simulink model "projeto_SOGI_PLL"  (R2018a)
settings: Solver=ode4  StartTime=0.0  StopTime=1  FixedStep=1e-4  RelTol=1e-3
undefined symbols (not defined in the file): Ibase, L, R, Vdc, Vp
libraries: powerlib_meascontrol x3, peTransforms x1
settings Model: Creator=lucas.figueiredo  LastModifiedBy=lucas.figueiredo

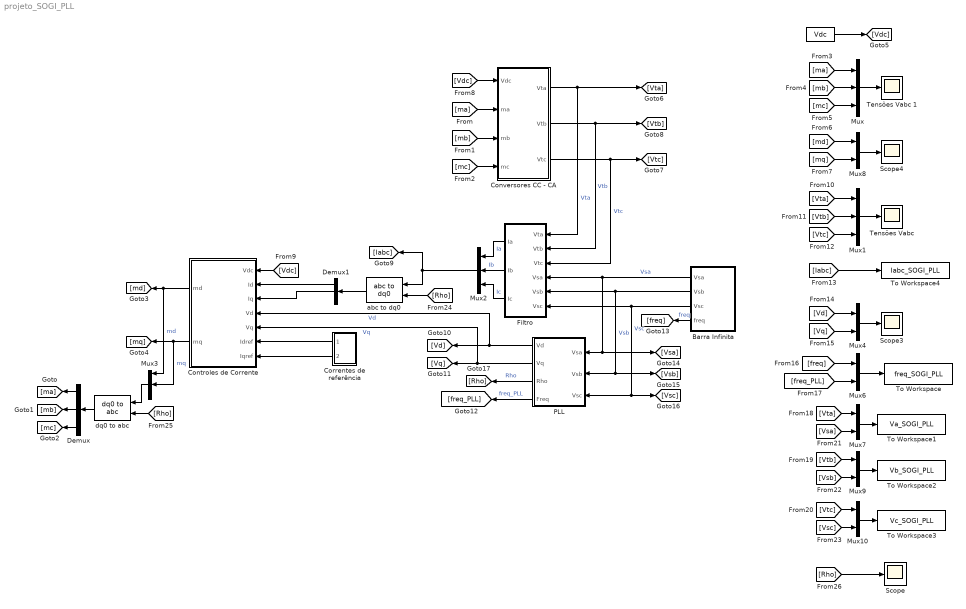
== system projeto_SOGI_PLL ==
  " " : Constant  Value=Vdc
  Barra Infinita : Subsystem
  Controles de Corrente : Subsystem
  Conversores CC - CA : Subsystem
  Correntes de referência : Subsystem
  Demux : Demux  Outputs=3
  Demux1 : Demux  Outputs=3
  Filtro : Subsystem
  Mux{,1..3} (4 alike) : Mux  Inputs=3
  Mux{4,6..10} (6 alike) : Mux  Inputs=2
  PLL : Subsystem
  Scope : Scope
  Scope3 : Scope
  Scope4 : Scope
  Tensões Vabc : Scope
  Tensões Vabc 1 : Scope
  To Workspace : ToWorkspace  VariableName=freq_SOGI_PLL  SaveFormat=Structure With Time  SampleTime=-1
      settings: Save2DSignal=2-D array (concatenate along first dimension)
  To Workspace1 : ToWorkspace  VariableName=Va_SOGI_PLL  SaveFormat=Structure With Time  SampleTime=-1
      settings: Save2DSignal=2-D array (concatenate along first dimension)
  To Workspace2 : ToWorkspace  VariableName=Vb_SOGI_PLL  SaveFormat=Structure With Time  SampleTime=-1
      settings: Save2DSignal=2-D array (concatenate along first dimension)
  To Workspace3 : ToWorkspace  VariableName=Vc_SOGI_PLL  SaveFormat=Structure With Time  SampleTime=-1
      settings: Save2DSignal=2-D array (concatenate along first dimension)
  To Workspace4 : ToWorkspace  VariableName=Iabc_SOGI_PLL  SaveFormat=Structure With Time  SampleTime=-1
      settings: Save2DSignal=2-D array (concatenate along first dimension)
  abc to dq0 : powerlib_meascontrol/Transformations/abc to dq0  Alignment=90 degrees behind phase A axis
  dq0 to abc : powerlib_meascontrol/Transformations/dq0 to abc  Alignment=90 degrees behind phase A axis
  wires:
  Mux/1 -> Tensões Vabc 1/1
  Mux1/1 -> Tensões Vabc/1
  Conversores CC - CA/1(Vta) -> Filtro/1(Vta), [Vta]  "Vta"
  Conversores CC - CA/2(Vtb) -> Filtro/2(Vtb), [Vtb]  "Vtb"
  Conversores CC - CA/3("Vtc ") -> Filtro/3(Vtc), [Vtc]  "Vtc"
  Filtro/1(Ia) -> Mux2/1  "Ia"
  Filtro/2(Ib) -> Mux2/2  "Ib"
  Filtro/3(Ic) -> Mux2/3  "Ic"
  Mux2/1 -> [Iabc], abc to dq0/1
  Mux3/1 -> dq0 to abc/1
  dq0 to abc/1 -> Demux/1
  Barra Infinita/1(Vsa) -> [Vsa], PLL/1(Vsa), Filtro/4(Vsa)  "Vsa"
  Barra Infinita/2(Vsb) -> [Vsb], PLL/2(Vsb), Filtro/5(Vsb)  "Vsb"
  Barra Infinita/3(Vsc) -> [Vsc], PLL/3(Vsc), Filtro/6(Vsc)  "Vsc"
  PLL/1(Vd) -> [Vd], Controles de Corrente/4(Vd)  "Vd"
  PLL/2(Vq) -> [Vq], Controles de Corrente/5(Vq)  "Vq"
  abc to dq0/1 -> Demux1/1
  Demux1/1 -> Controles de Corrente/2(Id)
  Demux1/2 -> Controles de Corrente/3(Iq)
  Controles de Corrente/1(md) -> [md], Mux3/1  "md"
  Controles de Corrente/2(mq) -> [mq], Mux3/2  "mq"
  [ma] -> Conversores CC - CA/2(ma)
  [mb] -> Conversores CC - CA/3(mb)
  [mc] -> Conversores CC - CA/4(mc)
  Demux/1 -> [ma]
  Demux/2 -> [mb]
  Demux/3 -> [mc]
  [ma] -> Mux/1
  [mb] -> Mux/2
  [mc] -> Mux/3
  Mux8/1 -> Scope4/1
  [md] -> Mux8/1
  [mq] -> Mux8/2
  " "/1 -> [Vdc]
  [Vdc] -> Conversores CC - CA/1("Vdc ")
  [Vdc] -> Controles de Corrente/1(Vdc)
  [Vta] -> Mux1/1
  [Vtb] -> Mux1/2
  [Vtc] -> Mux1/3
  [Iabc] -> To Workspace4/1
  Mux4/1 -> Scope3/1
  [Vq] -> Mux4/2
  [Vd] -> Mux4/1
  [freq] -> Mux6/1
  Mux6/1 -> To Workspace/1
  PLL/4(Freq) -> [freq_PLL]  "freq_PLL"
  Barra Infinita/4(freq) -> [freq]  "freq"
  [Vta] -> Mux7/1
  [Vtb] -> Mux9/1
  [Vtc] -> Mux10/1
  [Vsa] -> Mux7/2
  [Vsb] -> Mux9/2
  [Vsc] -> Mux10/2
  [freq_PLL] -> Mux6/2
  PLL/3(Rho) -> [Rho]  "Rho"
  [Rho] -> abc to dq0/2
  [Rho] -> dq0 to abc/2
  Correntes de referência/1(Idref) -> Controles de Corrente/6(Idref)
  Correntes de referência/2(Iqref) -> Controles de Corrente/7(Iqref)
  [Rho] -> Scope/1
  Mux7/1 -> To Workspace1/1
  Mux9/1 -> To Workspace2/1
  Mux10/1 -> To Workspace3/1

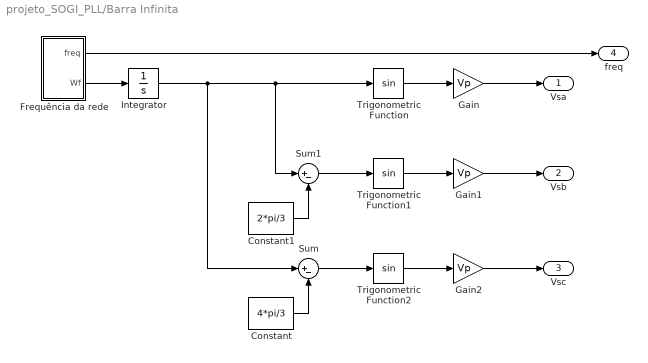
== system projeto_SOGI_PLL/Barra Infinita ==
  Constant : Constant  Value=4*pi/3
  Constant1 : Constant  Value=2*pi/3
  Frequência da rede : Subsystem
  Gain : Gain  Gain=Vp
  Gain1 : Gain  Gain=Vp
  Gain2 : Gain  Gain=Vp
  Integrator : Integrator
  Sum : Sum  Inputs=|+-
  Sum1 : Sum  Inputs=|+-
  Trigonometric Function : Trigonometry
  Trigonometric Function1 : Trigonometry
  Trigonometric Function2 : Trigonometry
  Vsa : Outport
  Vsb : Outport  Port=2
  Vsc : Outport  Port=3
  freq : Outport  Port=4
  wires:
  Integrator/1 -> Sum/1, Sum1/1, Trigonometric Function/1
  Frequência da rede/2(Wf) -> Integrator/1
  Constant/1 -> Sum/2
  Frequência da rede/1(freq) -> freq/1
  Sum/1 -> Trigonometric Function2/1
  Sum1/1 -> Trigonometric Function1/1
  Constant1/1 -> Sum1/2
  Trigonometric Function/1 -> Gain/1
  Trigonometric Function1/1 -> Gain1/1
  Trigonometric Function2/1 -> Gain2/1
  Gain/1 -> Vsa/1
  Gain1/1 -> Vsb/1
  Gain2/1 -> Vsc/1

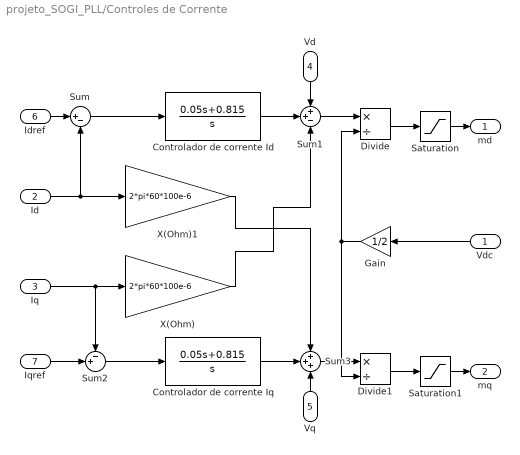
== system projeto_SOGI_PLL/Controles de Corrente ==
  Vdc : Inport
  Id : Inport  Port=2
  Iq : Inport  Port=3
  Vd : Inport  Port=4
  Vq : Inport  Port=5
  Idref : Inport  Port=6
  Iqref : Inport  Port=7
  Controlador de corrente Id : TransferFcn  Numerator=[0.05 0.815]  Denominator=[1 0]
  Controlador de corrente Iq : TransferFcn  Numerator=[0.05 0.815]  Denominator=[1 0]
  Divide : Product  Inputs=*/
  Divide1 : Product  Inputs=*/
  Gain : Gain  Gain=1/2
  Saturation : Saturate  UpperLimit=1  LowerLimit=-1
  Saturation1 : Saturate  UpperLimit=1  LowerLimit=-1
  Sum : Sum  Inputs=|+-
  Sum1 : Sum  Inputs=++-
  Sum2 : Sum  Inputs=-+|
  Sum3 : Sum  Inputs=+++
  X(Ohm) : Gain  Gain=2*pi*60*100e-6
  X(Ohm)1 : Gain  Gain=2*pi*60*100e-6
  md : Outport
  mq : Outport  Port=2
  wires:
  Sum2/1 -> Controlador de corrente Iq/1
  Divide1/1 -> Saturation1/1
  Divide/1 -> Saturation/1
  Controlador de corrente Id/1 -> Sum1/2
  Sum3/1 -> Divide1/1
  X(Ohm)1/1 -> Sum3/1
  Iqref/1 -> Sum2/2
  Gain/1 -> Divide1/2, Divide/2
  Controlador de corrente Iq/1 -> Sum3/2
  Sum/1 -> Controlador de corrente Id/1
  Sum1/1 -> Divide/1
  X(Ohm)/1 -> Sum1/3
  Vdc/1 -> Gain/1
  Vq/1 -> Sum3/3
  Vd/1 -> Sum1/1
  Iq/1 -> Sum2/1, X(Ohm)/1
  Id/1 -> Sum/2, X(Ohm)1/1
  Saturation1/1 -> mq/1
  Saturation/1 -> md/1
  Idref/1 -> Sum/1

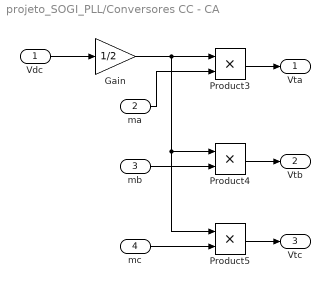
== system projeto_SOGI_PLL/Conversores CC - CA ==
  "Vdc " : Inport
  ma : Inport  Port=2
  mb : Inport  Port=3
  mc : Inport  Port=4
  Gain : Gain  Gain=1/2
  Product3 : Product
  Product4 : Product
  Product5 : Product
  Vta : Outport
  Vtb : Outport  Port=2
  "Vtc " : Outport  Port=3
  wires:
  ma/1 -> Product3/2
  mb/1 -> Product4/2
  Product3/1 -> Vta/1
  Gain/1 -> Product4/1, Product5/1, Product3/1
  Product5/1 -> "Vtc "/1
  Product4/1 -> Vtb/1
  "Vdc "/1 -> Gain/1
  mc/1 -> Product5/2

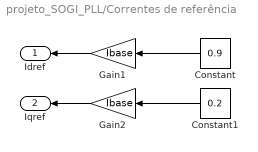
== system projeto_SOGI_PLL/Correntes de referência ==
  Constant : Constant  Value=0.9
  Constant1 : Constant  Value=0.2
  Gain1 : Gain  Gain=Ibase
  Gain2 : Gain  Gain=Ibase
  Idref : Outport
  Iqref : Outport  Port=2
  wires:
  Constant1/1 -> Gain2/1
  Constant/1 -> Gain1/1
  Gain2/1 -> Iqref/1
  Gain1/1 -> Idref/1

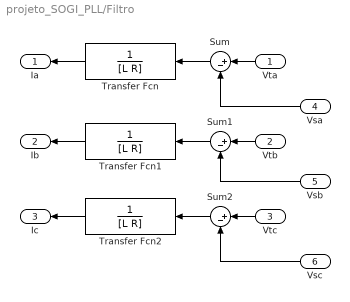
== system projeto_SOGI_PLL/Filtro ==
  Vta : Inport
  Vtb : Inport  Port=2
  Vtc : Inport  Port=3
  Vsa : Inport  Port=4
  Vsb : Inport  Port=5
  Vsc : Inport  Port=6
  Sum : Sum  Inputs=|+-
  Sum1 : Sum  Inputs=|+-
  Sum2 : Sum  Inputs=|+-
  Transfer Fcn : TransferFcn  Denominator=[L R]
  Transfer Fcn1 : TransferFcn  Denominator=[L R]
  Transfer Fcn2 : TransferFcn  Denominator=[L R]
  Ia : Outport
  Ib : Outport  Port=2
  Ic : Outport  Port=3
  wires:
  Transfer Fcn1/1 -> Ib/1
  Vtc/1 -> Sum2/1
  Transfer Fcn2/1 -> Ic/1
  Transfer Fcn/1 -> Ia/1
  Sum/1 -> Transfer Fcn/1
  Vta/1 -> Sum/1
  Vsa/1 -> Sum/2
  Sum2/1 -> Transfer Fcn2/1
  Sum1/1 -> Transfer Fcn1/1
  Vtb/1 -> Sum1/1
  Vsc/1 -> Sum2/2
  Vsb/1 -> Sum1/2

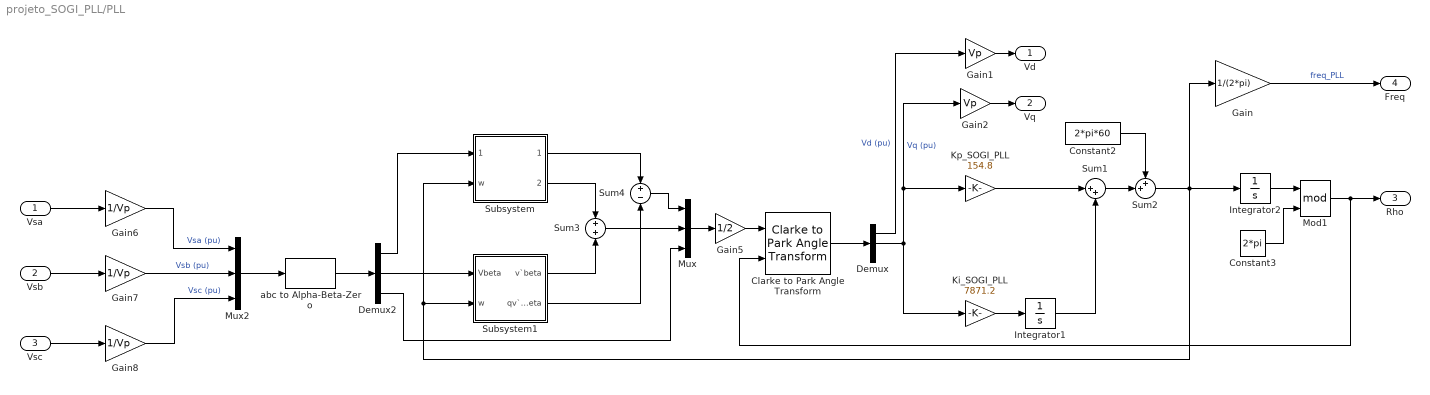
== system projeto_SOGI_PLL/PLL ==
  Vsa : Inport
  Vsb : Inport  Port=2
  Vsc : Inport  Port=3
  Clarke to Park Angle Transform : peTransforms/Clarke to Park Angle Transform  AxisAlignment=Q-axis
  Constant2 : Constant  Value=2*pi*60
  Constant3 : Constant  Value=2*pi
  Demux : Demux  Outputs=3
  Demux2 : Demux  Outputs=3
  Gain : Gain  Gain=1/(2*pi)
  Gain1 : Gain  Gain=Vp
  Gain2 : Gain  Gain=Vp
  Gain5 : Gain  Gain=1/2
  Gain6 : Gain  Gain=1/Vp
  Gain7 : Gain  Gain=1/Vp
  Gain8 : Gain  Gain=1/Vp
  Integrator1 : Integrator
  Integrator2 : Integrator
  Ki_SOGI_PLL : Gain  Gain=7871.2
  Kp_SOGI_PLL : Gain  Gain=154.8
  Mod1 : Math  Operator=mod  SaturateOnIntegerOverflow=on
  Mux : Mux  Inputs=3
  Mux2 : Mux  Inputs=3
  Subsystem : Subsystem
  Subsystem1 : Subsystem
  Sum1 : Sum  Inputs=|++
  Sum2 : Sum  Inputs=++|
  Sum3 : Sum  Inputs=+|+
  Sum4 : Sum  Inputs=+|-
  abc to Alpha-Beta-Zero : powerlib_meascontrol/Transformations/abc to Alpha-Beta-Zero
      settings: SourceProductName=Simscape Power Systems
  Vd : Outport
  Vq : Outport  Port=2
  Rho : Outport  Port=3
  Freq : Outport  Port=4
  wires:
  Subsystem/1(v`alpha) -> Sum4/1
  Subsystem1/2(qv`beta) -> Sum4/2
  Kp_SOGI_PLL/1 -> Sum1/1
  Subsystem1/1(v`beta) -> Sum3/2
  Sum4/1 -> Mux/1
  Demux2/3 -> Mux/3
  Sum2/1 -> Gain/1, Subsystem1/2(w), Subsystem/2(w), Integrator2/1
  Constant2/1 -> Sum2/1
  Mod1/1 -> Rho/1, Clarke to Park Angle Transform/2
  Demux/2 -> Ki_SOGI_PLL/1, Gain2/1, Kp_SOGI_PLL/1  "Vq (pu)"
  Sum3/1 -> Mux/2
  Demux2/1 -> Subsystem/1(Valpha)
  abc to Alpha-Beta-Zero/1 -> Demux2/1
  Constant3/1 -> Mod1/2
  Mux/1 -> Gain5/1
  Sum1/1 -> Sum2/2
  Integrator1/1 -> Sum1/2
  Mux2/1 -> abc to Alpha-Beta-Zero/1
  Gain5/1 -> Clarke to Park Angle Transform/1
  Clarke to Park Angle Transform/1 -> Demux/1
  Demux2/2 -> Subsystem1/1(Vbeta)
  Ki_SOGI_PLL/1 -> Integrator1/1
  Subsystem/2(qv`alpha) -> Sum3/1
  Integrator2/1 -> Mod1/1
  Gain6/1 -> Mux2/1  "Vsa (pu)"
  Vsc/1 -> Gain8/1
  Gain7/1 -> Mux2/2  "Vsb (pu)"
  Gain8/1 -> Mux2/3  "Vsc (pu)"
  Vsb/1 -> Gain7/1
  Vsa/1 -> Gain6/1
  Gain/1 -> Freq/1  "freq_PLL"
  Demux/1 -> Gain1/1  "Vd (pu)"
  Gain1/1 -> Vd/1
  Gain2/1 -> Vq/1

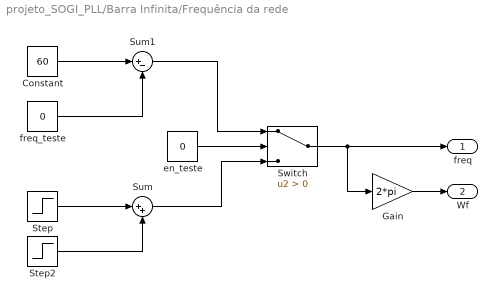
== system projeto_SOGI_PLL/Barra Infinita/Frequência da rede ==
  Constant : Constant  Value=60
  Gain : Gain  Gain=2*pi
  Step : Step  Time=0.2  Before=60  After=50  SampleTime=0
  Step2 : Step  Time=0.4  After=10  SampleTime=0
  Sum : Sum  Inputs=|++
  Sum1 : Sum  Inputs=|+-
  Switch : Switch  Criteria=u2 > Threshold
  en_teste : Constant  Value=0
  freq_teste : Constant  Value=0
  freq : Outport
  Wf : Outport  Port=2
  wires:
  Switch/1 -> Gain/1, freq/1
  Gain/1 -> Wf/1
  en_teste/1 -> Switch/2
  Step2/1 -> Sum/2
  Sum/1 -> Switch/3
  Sum1/1 -> Switch/1
  Step/1 -> Sum/1
  Constant/1 -> Sum1/1
  freq_teste/1 -> Sum1/2

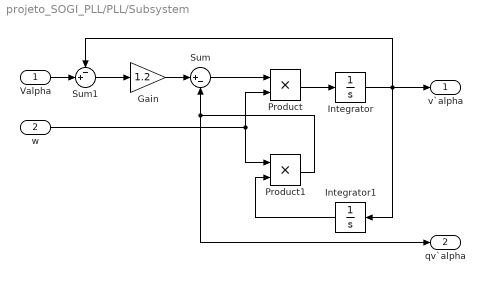
== system projeto_SOGI_PLL/PLL/Subsystem ==
  Valpha : Inport
  w : Inport  Port=2
  Gain : Gain  Gain=1.2
  Integrator : Integrator
  Integrator1 : Integrator
  Product : Product
  Product1 : Product
  Sum : Sum  Inputs=|+-
  Sum1 : Sum  Inputs=-+|
  v`alpha : Outport
  qv`alpha : Outport  Port=2
  wires:
  Gain/1 -> Sum/1
  Sum/1 -> Product/1
  w/1 -> Product1/1, Product/2
  Product/1 -> Integrator/1
  Integrator/1 -> v`alpha/1, Sum1/1, Integrator1/1
  Product1/1 -> qv`alpha/1, Sum/2
  Integrator1/1 -> Product1/2
  Valpha/1 -> Sum1/2
  Sum1/1 -> Gain/1

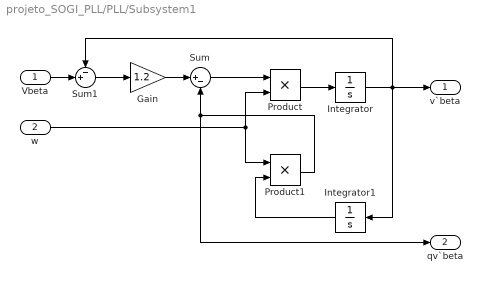
== system projeto_SOGI_PLL/PLL/Subsystem1 ==
  Vbeta : Inport
  w : Inport  Port=2
  Gain : Gain  Gain=1.2
  Integrator : Integrator
  Integrator1 : Integrator
  Product : Product
  Product1 : Product
  Sum : Sum  Inputs=|+-
  Sum1 : Sum  Inputs=-+|
  v`beta : Outport
  qv`beta : Outport  Port=2
  wires:
  Integrator1/1 -> Product1/2
  Product1/1 -> qv`beta/1, Sum/2
  Vbeta/1 -> Sum1/2
  Product/1 -> Integrator/1
  Integrator/1 -> v`beta/1, Sum1/1, Integrator1/1
  w/1 -> Product1/1, Product/2
  Sum/1 -> Product/1
  Gain/1 -> Sum/1
  Sum1/1 -> Gain/1
